simulink model "circuitss"  (Simulink 7.4)
settings: Solver=ode45  StartTime=0.0  StopTime=10.0  RelTol=1e-3
values from neighbouring files (symbols this model uses):
  C = [1 0; 0 1; 1 -R; 0 R; 0 -1]    [ssmodels.m]
  L = 1    [ssmodels.m]
  R = 1    [ssmodels.m]
settings Model: Creator=eechris  LastModifiedBy=eechris

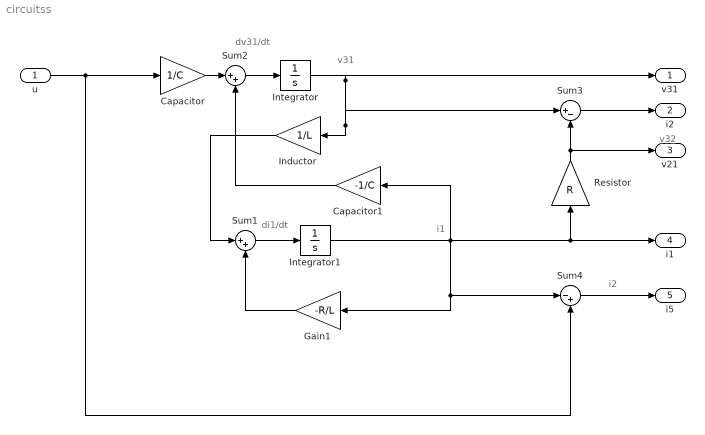
== system circuitss ==
  note: dv31/dt
  note: v31
  note: v32
  note: di1/dt
  note: i1
  note: i2
  u : Inport  OutDataType=fixdt(1, 16)  OutScaling=2^0
  Capacitor : Gain  Gain=1/C  ParameterDataType=fixdt(1, 16)  ParameterScaling=2^0  OutDataType=fixdt(1, 16)  OutScaling=2^0
  Capacitor1 : Gain  Gain=-1/C  ParameterDataType=fixdt(1, 16)  ParameterScaling=2^0  OutDataType=fixdt(1, 16)  OutScaling=2^0
  Gain1 : Gain  Gain=-R/L  ParameterDataType=fixdt(1, 16)  ParameterScaling=2^0  OutDataType=fixdt(1, 16)  OutScaling=2^0
  Inductor : Gain  Gain=1/L  ParameterDataType=fixdt(1, 16)  ParameterScaling=2^0  OutDataType=fixdt(1, 16)  OutScaling=2^0
  Integrator : Integrator
  Integrator1 : Integrator
  Resistor : Gain  Gain=R  ParameterDataType=fixdt(1, 16)  ParameterScaling=2^0  OutDataType=fixdt(1, 16)  OutScaling=2^0
  Sum1 : Sum  Inputs=|++  OutDataType=fixdt(1, 16)  OutScaling=2^0
  Sum2 : Sum  Inputs=|++  OutDataType=fixdt(1, 16)  OutScaling=2^0
  Sum3 : Sum  Inputs=|+-  OutDataType=fixdt(1, 16)  OutScaling=2^0
  Sum4 : Sum  Inputs=|-+  OutDataType=fixdt(1, 16)  OutScaling=2^0
  v31 : Outport  OutDataType=fixdt(1, 16)  OutScaling=2^0
  i2 : Outport  Port=2  OutDataType=fixdt(1, 16)  OutScaling=2^0
  v21 : Outport  Port=3  OutDataType=fixdt(1, 16)  OutScaling=2^0
  i1 : Outport  Port=4  OutDataType=fixdt(1, 16)  OutScaling=2^0
  i5 : Outport  Port=5  OutDataType=fixdt(1, 16)  OutScaling=2^0
  wires:
  Integrator/1 -> v31/1, Inductor/1, Sum3/1
  Capacitor/1 -> Sum2/1
  Sum2/1 -> Integrator/1
  Inductor/1 -> Sum1/1
  Sum1/1 -> Integrator1/1
  Gain1/1 -> Sum1/2
  Capacitor1/1 -> Sum2/2
  u/1 -> Capacitor/1, Sum4/2
  Resistor/1 -> Sum3/2, v21/1
  Sum3/1 -> i2/1
  Integrator1/1 -> Capacitor1/1, i1/1, Resistor/1, Gain1/1, Sum4/1
  Sum4/1 -> i5/1
